simulink model "configure2pressure"  (R2025a)
settings: Solver=VariableStepAuto  StartTime=0.0  StopTime=10.0  RelTol=1e-3
settings Model: Creator=dperera  LastModifiedBy=dperera

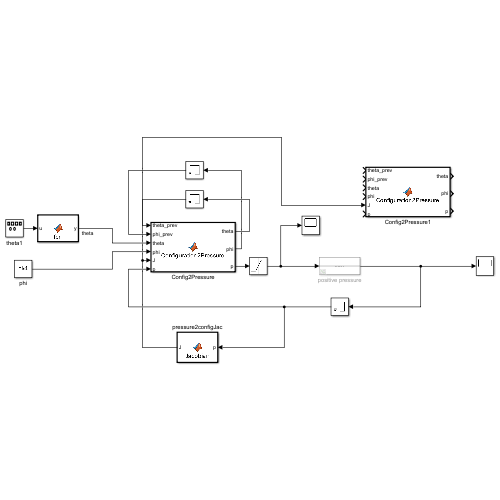
[thumbnail: Simulink's stored preview of the top-level diagram]
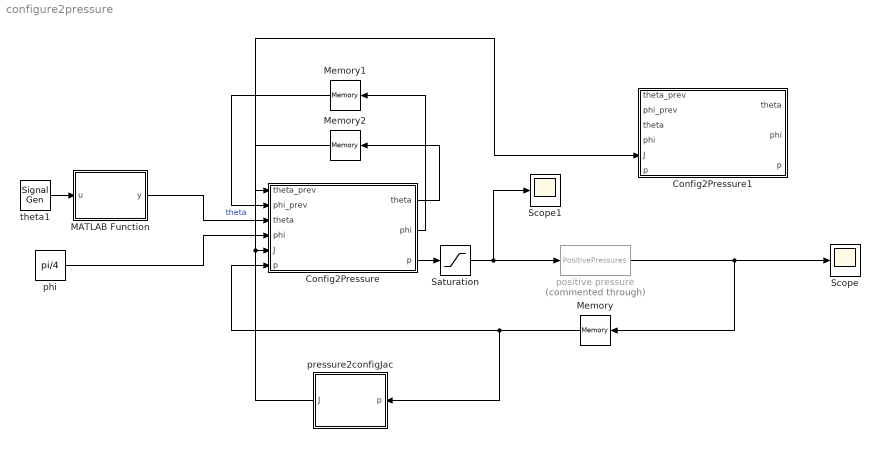
== system configure2pressure ==
  Config2Pressure : MATLAB Function  TreatAsAtomicUnit=on
  Config2Pressure1 : MATLAB Function  TreatAsAtomicUnit=on
  MATLAB Function : MATLAB Function  TreatAsAtomicUnit=on
  Memory : Memory  InitialCondition=[1.0;0.0;-1.0]  InheritSampleTime=on
  Memory1 : Memory  InheritSampleTime=on
  Memory2 : Memory  InheritSampleTime=on
  Saturation : Saturate  UpperLimit=300000  LowerLimit=-300000
  Scope : Scope
      settings: ActiveDisplayYMinimum=-37499.999999999993  ActiveDisplayYMaximum=337500
  Scope1 : Scope
      settings: ActiveDisplayYMinimum=-6484.0279388846739  ActiveDisplayYMaximum=6484.0279388846739
  phi : Constant  Value=pi/4
  positive pressure : MATLABFcn  Commented=through  MATLABFcn=PositivePressures  OutputDimensions=[3,1]  Output1D=off
  pressure2configJac : MATLAB Function  TreatAsAtomicUnit=on
  theta1 : SignalGenerator  WaveForm=sawtooth  Amplitude=pi  Frequency=0.5*2*pi  Units=rad/sec  VectorParams1D=off
  wires:
  theta1/1 -> MATLAB Function/1(u)
  MATLAB Function/1(y) -> Config2Pressure/3("theta ")  "theta"
  phi/1 -> Config2Pressure/4("phi ")
  Config2Pressure/3(p) -> Saturation/1
  Memory/1 -> pressure2configJac/1(p), Config2Pressure/6("p ")
  positive pressure/1 -> Scope/1, Memory/1
  pressure2configJac/1(J) -> Config2Pressure/5(J), Config2Pressure1/5(J)
  Saturation/1 -> Scope1/1, positive pressure/1
  Config2Pressure/1(theta) -> Memory2/1
  Memory2/1 -> Config2Pressure/1(theta_prev)
  Config2Pressure/2(phi) -> Memory1/1
  Memory1/1 -> Config2Pressure/2(phi_prev)

== matlab function configure2pressure/pressure2configJac ==
  data: J output; p input
function J = Jacobian(p)

r = 0.013;
K = 0.0155;
A = pi*(0.013/2)^2;

J = pressure2configJacobian(p, r, K, A);

end

== matlab function configure2pressure/Config2Pressure ==
  data: theta_prev input; phi_prev input; theta output; phi output; theta input; p output; phi input; J input; p input
function [theta, phi, p] = Configuration2Pressure(theta_prev, phi_prev, theta, phi, J, p)

% persistent theta_prev phi_prev;
% 
% if isempty(theta_prev)
%     theta_prev = 0.0;
% end
% 
% if isempty(phi_prev)
%     phi_prev = 0.0;
% end

dp = J \ ([theta; phi]-[theta_prev; phi_prev]);

% theta_prev = theta;
% phi_prev = phi;

p = reshape(p,[3,1]);
p = p + [-(dp(1)+dp(2)); dp(1); dp(2)];

end

== matlab function configure2pressure/Config2Pressure1 ==
  data: theta_prev input; phi_prev input; theta output; phi output; theta input; p output; phi input; J input; p input
function [theta, phi, p] = Configuration2Pressure(theta_prev, phi_prev, theta, phi, J, p)

% persistent theta_prev phi_prev;
% 
% if isempty(theta_prev)
%     theta_prev = 0.0;
% end
% 
% if isempty(phi_prev)
%     phi_prev = 0.0;
% end

dp = J \ ([theta; phi]-[theta_prev; phi_prev]);

% theta_prev = theta;
% phi_prev = phi;

p = reshape(p,[3,1]);
p = p + [-(dp(1)+dp(2)); dp(1); dp(2)];

end

== matlab function configure2pressure/MATLAB Function ==
  data: u input; y output
function y = fcn(u)

y = wrapToPi(u - pi);
